simulink model "sampleModel20"  (R2021a)
settings: Solver=VariableStepAuto  StartTime=0.0  StopTime=10.0  RelTol=1e-3
undefined symbols (not defined in the file): DiscIntNeverNeededParam, magnitude, Newton, Raphson
libraries: simulink x274, pid_lib x17
(part 8 of 16)

== system sampleModel20/cfblk97/cfblk4/cfblk4 ==
  cfblk1 : Inport
  cfblk14 : Inport  Port=2
  cfblk15 : Inport  Port=3
  cfblk16 : Inport  Port=4
  cfblk17 : Inport  Port=5
  cfblk10 : Subsystem
  cfblk11 : Subsystem
  cfblk12 : Subsystem
  cfblk13 : Subsystem
  cfblk{18..23} (6 alike) : Delay  SampleTime=1
  cfblk3 : Trigonometry
  cfblk4 : ComplexToMagnitudeAngle
  cfblk5 : simulink/Math Operations/Slider Gain  gain=1  low=0  high=2
  cfblk6 : simulink/Math Operations/Slider Gain  gain=1  low=0  high=2
  cfblk7 : Abs
  cfblk8 : Subsystem
  cfblk9 : Subsystem
  cfblk2 : Outport
  wires:
  cfblk1/1 -> cfblk7/1, cfblk12/4(cfblk7)
  cfblk6/1 -> cfblk10/1(cfblk1)
  cfblk4/1 -> cfblk8/1(cfblk1)
  cfblk4/2 -> cfblk6/1, cfblk10/5(cfblk10), cfblk11/5(cfblk9), cfblk11/9(cfblk13), cfblk10/7(cfblk12)
  cfblk7/1 -> cfblk5/1, cfblk10/6(cfblk11), cfblk11/7(cfblk11), cfblk9/3(cfblk6), cfblk11/10(cfblk14)
  cfblk16/1 -> cfblk2/1
  cfblk11/1(cfblk2) -> cfblk13/2(cfblk12)
  cfblk12/1(cfblk2) -> cfblk11/1(cfblk1)
  cfblk10/1(cfblk2) -> cfblk18/1, cfblk19/1
  cfblk3/1 -> cfblk11/2(cfblk6), cfblk9/7(cfblk10)
  cfblk15/1 -> cfblk8/2(cfblk6)
  cfblk12/2(cfblk9) -> cfblk4/1
  cfblk5/1 -> cfblk12/2(cfblk5), cfblk9/4(cfblk7)
  cfblk17/1 -> cfblk10/2(cfblk7), cfblk11/6(cfblk10), cfblk13/3(cfblk13), cfblk13/5(cfblk15)
  cfblk14/1 -> cfblk9/1(cfblk1), cfblk13/6(cfblk16), cfblk9/6(cfblk9)
  cfblk13/1(cfblk2) -> cfblk10/3(cfblk8)
  cfblk13/2(cfblk17) -> cfblk9/5(cfblk8), cfblk20/1
  cfblk8/1(cfblk2) -> cfblk9/2(cfblk5)
  cfblk8/2(cfblk7) -> cfblk3/1, cfblk13/4(cfblk14), cfblk11/8(cfblk12)
  cfblk9/3(cfblk12) -> cfblk10/4(cfblk9)
  cfblk18/1 -> cfblk12/1(cfblk1)
  cfblk19/1 -> cfblk12/5(cfblk8)
  cfblk20/1 -> cfblk11/4(cfblk8)
  cfblk9/1(cfblk2) -> cfblk21/1
  cfblk21/1 -> cfblk13/1(cfblk1)
  cfblk9/2(cfblk11) -> cfblk22/1
  cfblk22/1 -> cfblk11/3(cfblk7)
  cfblk9/4(cfblk13) -> cfblk23/1
  cfblk23/1 -> cfblk12/3(cfblk6)

== system sampleModel20/cfblk97/cfblk4/cfblk5 ==
  cfblk1 : Inport
  cfblk7 : Inport  Port=2
  cfblk8 : Inport  Port=3
  cfblk9 : Inport  Port=4
  cfblk10 : Inport  Port=5
  cfblk11 : Inport  Port=6
  cfblk12 : Inport  Port=7
  cfblk13 : Inport  Port=8
  cfblk14 : Inport  Port=9
  cfblk15 : Inport  Port=10
  cfblk3 : Rounding
  cfblk4 : MinMax  Inputs=2
  cfblk5 : Sum  Inputs=+-
  cfblk6 : Abs
  cfblk2 : Outport
  cfblk16 : Outport  Port=2
  cfblk17 : Outport  Port=3
  wires:
  cfblk7/1 -> cfblk6/1
  cfblk12/1 -> cfblk3/1
  cfblk6/1 -> cfblk5/1
  cfblk13/1 -> cfblk17/1
  cfblk10/1 -> cfblk5/2
  cfblk1/1 -> cfblk4/1
  cfblk11/1 -> cfblk2/1
  cfblk3/1 -> cfblk4/2
  cfblk4/1 -> cfblk16/1

== system sampleModel20/cfblk97/cfblk4/cfblk6 ==
  cfblk1 : Inport
  cfblk9 : Inport  Port=2
  cfblk{12..16} (5 alike) : Delay  SampleTime=1
  cfblk3 : Abs
  cfblk4 : Abs
  cfblk5 : simulink/Math Operations/MinMax Running Resettable  Function=min  vinit=0.0
  cfblk6 : Constant  Value=[-933538233.402793]  SampleTime=1
  cfblk7 : Subsystem
  cfblk8 : Subsystem
  cfblk2 : Outport
  cfblk10 : Outport  Port=2
  cfblk11 : Outport  Port=3
  wires:
  cfblk3/1 -> cfblk8/1(cfblk1), cfblk8/5(cfblk11)
  cfblk8/2(cfblk15) -> cfblk2/1
  cfblk6/1 -> cfblk5/1
  cfblk4/1 -> cfblk8/2(cfblk8), cfblk5/2, cfblk15/1, cfblk16/1
  cfblk7/1(cfblk2) -> cfblk8/3(cfblk9)
  cfblk7/2(cfblk13) -> cfblk3/1
  cfblk7/3(cfblk14) -> cfblk10/1
  cfblk5/1 -> cfblk8/6(cfblk12), cfblk8/7(cfblk13), cfblk8/8(cfblk14), cfblk13/1, cfblk14/1
  cfblk7/4(cfblk15) -> cfblk4/1
  cfblk9/1 -> cfblk8/4(cfblk10), cfblk7/5(cfblk10)
  cfblk1/1 -> cfblk7/3(cfblk8)
  cfblk7/5(cfblk16) -> cfblk11/1
  cfblk8/1(cfblk2) -> cfblk12/1
  cfblk12/1 -> cfblk7/1(cfblk1)
  cfblk13/1 -> cfblk7/2(cfblk7)
  cfblk14/1 -> cfblk7/7(cfblk12)
  cfblk15/1 -> cfblk7/4(cfblk9)
  cfblk16/1 -> cfblk7/6(cfblk11)

== system sampleModel20/cfblk100/cfblk11/cfblk7/cfblk4 ==
  cfblk1 : Inport
  cfblk9 : Inport  Port=2
  cfblk10 : Inport  Port=3
  cfblk11 : Inport  Port=4
  cfblk12 : Inport  Port=5
  cfblk13 : Inport  Port=6
  cfblk14 : Inport  Port=7
  cfblk15 : Inport  Port=8
  cfblk3 : Math  Operator=magnitude^2  SaturateOnIntegerOverflow=on
  cfblk4 : ComplexToRealImag
  cfblk5 : Gain  Gain=[-735360419.453945]
  cfblk6 : ComplexToMagnitudeAngle
  cfblk7 : MinMax
  cfblk8 : Sum  Inputs=+
  cfblk2 : Outport
  cfblk16 : Outport  Port=2
  cfblk17 : Outport  Port=3
  wires:
  cfblk14/1 -> cfblk7/1
  cfblk8/1 -> cfblk6/1
  cfblk15/1 -> cfblk16/1
  cfblk3/1 -> cfblk4/1
  cfblk13/1 -> cfblk17/1
  cfblk12/1 -> cfblk2/1
  cfblk9/1 -> cfblk5/1
  cfblk1/1 -> cfblk8/1
  cfblk6/1 -> cfblk3/1

== system sampleModel20/cfblk100/cfblk11/cfblk7/cfblk5 ==
  cfblk1 : Inport
  cfblk6 : Inport  Port=2
  cfblk7 : Inport  Port=3
  cfblk3 : Sum  Inputs=|++
  cfblk4 : simulink/Math Operations/MinMax Running Resettable  Function=min  vinit=0.0
  cfblk5 : MinMax
  cfblk2 : Outport
  cfblk8 : Outport  Port=2
  cfblk9 : Outport  Port=3
  cfblk10 : Outport  Port=4
  wires:
  cfblk3/1 -> cfblk2/1, cfblk4/1
  cfblk5/1 -> cfblk10/1
  cfblk4/1 -> cfblk5/1
  cfblk6/1 -> cfblk8/1, cfblk3/2
  cfblk1/1 -> cfblk9/1
  cfblk7/1 -> cfblk3/1, cfblk4/2

== system sampleModel20/cfblk100/cfblk11/cfblk7/cfblk6 ==
  cfblk1 : Inport
  cfblk10 : Inport  Port=2
  cfblk11 : Inport  Port=3
  cfblk12 : Inport  Port=4
  cfblk13 : Inport  Port=5
  cfblk3 : simulink/Math Operations/MinMax Running Resettable  Function=min  vinit=0.0
  cfblk4 : simulink/Math Operations/Slider Gain  gain=1  low=0  high=2
  cfblk5 : Sin  TimeSource=Use external signal  SampleTime=0
  cfblk6 : Squeeze
  cfblk7 : DotProduct  InputSameDT=on  OutDataTypeStr=Inherit: Inherit via internal rule
  cfblk8 : MinMax  Function=max  Inputs=3
  cfblk9 : Abs
  cfblk2 : Outport
  cfblk14 : Outport  Port=2
  wires:
  cfblk10/1 -> cfblk5/1
  cfblk11/1 -> cfblk2/1
  cfblk9/1 -> cfblk6/1
  cfblk5/1 -> cfblk4/1, cfblk8/3
  cfblk1/1 -> cfblk8/1
  cfblk3/1 -> cfblk7/1
  cfblk7/1 -> cfblk14/1
  cfblk4/1 -> cfblk9/1
  cfblk13/1 -> cfblk3/1
  cfblk8/1 -> cfblk3/2
  cfblk12/1 -> cfblk8/2
  cfblk6/1 -> cfblk7/2

== system sampleModel20/cfblk100/cfblk11/cfblk8/cfblk12 ==
  cfblk1 : Inport
  cfblk10 : Inport  Port=2
  cfblk11 : Inport  Port=3
  cfblk12 : Inport  Port=4
  cfblk13 : Inport  Port=5
  cfblk14 : Inport  Port=6
  Action Port : ActionPort  ActionPortLabel=if(u1 >= 0)
  cfblk3 : Polyval  Coefs=[ +2.081618890e-019, -1.441693666e-014, +4.719686976e-010, -8.536869453e-006, +1.621573104e-001, -8.087801117e+001 ]
  cfblk4 : UnaryMinus
  cfblk5 : Product  Inputs=**
  cfblk6 : Sqrt  SaturateOnIntegerOverflow=on
  cfblk7 : simulink/Math Operations/Slider Gain  gain=1  low=0  high=2
  cfblk8 : MinMax  Function=max
  cfblk9 : Sum  Inputs=|++
  cfblk2 : Outport
  cfblk15 : Outport  Port=2
  cfblk16 : Outport  Port=3
  wires:
  cfblk9/1 -> cfblk5/1
  cfblk6/1 -> cfblk7/1
  cfblk5/1 -> cfblk15/1
  cfblk1/1 -> cfblk5/2
  cfblk11/1 -> cfblk2/1
  cfblk4/1 -> cfblk6/1
  cfblk14/1 -> cfblk3/1
  cfblk7/1 -> cfblk9/1
  cfblk3/1 -> cfblk4/1
  cfblk12/1 -> cfblk16/1
  cfblk8/1 -> cfblk9/2
  cfblk13/1 -> cfblk8/1

== system sampleModel20/cfblk100/cfblk11/cfblk8/cfblk13 ==
  cfblk1 : Inport
  cfblk4 : Inport  Port=2
  cfblk5 : Inport  Port=3
  cfblk6 : Inport  Port=4
  cfblk7 : Inport  Port=5
  cfblk8 : Inport  Port=6
  cfblk9 : Inport  Port=7
  Action Port : ActionPort  ActionPortLabel=else
  cfblk3 : Squeeze
  cfblk2 : Outport
  wires:
  cfblk9/1 -> cfblk2/1
  cfblk7/1 -> cfblk3/1

== system sampleModel20/cfblk100/cfblk11/cfblk8/cfblk5 ==
  cfblk1 : Inport
  cfblk5 : Inport  Port=2
  cfblk6 : Inport  Port=3
  cfblk7 : Inport  Port=4
  cfblk3 : Bias  Bias=[-726491726.571453]
  cfblk4 : DotProduct  InputSameDT=on  OutDataTypeStr=Inherit: Inherit via internal rule
  cfblk2 : Outport
  cfblk8 : Outport  Port=2
  wires:
  cfblk1/1 -> cfblk2/1
  cfblk7/1 -> cfblk3/1
  cfblk3/1 -> cfblk8/1
  cfblk5/1 -> cfblk4/1
  cfblk6/1 -> cfblk4/2

== system sampleModel20/cfblk100/cfblk11/cfblk8/cfblk6 ==
  cfblk1 : Inport
  cfblk6 : Inport  Port=2
  cfblk7 : Inport  Port=3
  cfblk8 : Inport  Port=4
  cfblk9 : Inport  Port=5
  cfblk10 : Inport  Port=6
  cfblk11 : Inport  Port=7
  cfblk12 : Inport  Port=8
  cfblk13 : Inport  Port=9
  cfblk3 : Bias  Bias=[914019764.906986]
  cfblk4 : Sqrt  SaturateOnIntegerOverflow=on
  cfblk5 : Reshape
  cfblk2 : Outport
  wires:
  cfblk3/1 -> cfblk5/1
  cfblk9/1 -> cfblk4/1
  cfblk10/1 -> cfblk2/1
  cfblk8/1 -> cfblk3/1

== system sampleModel20/cfblk100/cfblk11/cfblk8/cfblk7 ==
  cfblk1 : Inport
  cfblk8 : Inport  Port=2
  cfblk9 : Inport  Port=3
  cfblk10 : Inport  Port=4
  cfblk11 : Inport  Port=5
  cfblk12 : Inport  Port=6
  cfblk3 : Product  Inputs=*
  cfblk4 : DotProduct  InputSameDT=on  OutDataTypeStr=Inherit: Inherit via internal rule
  cfblk5 : PermuteDimensions
  cfblk6 : ComplexToMagnitudeAngle
  cfblk7 : Rounding
  cfblk2 : Outport
  cfblk13 : Outport  Port=2
  cfblk14 : Outport  Port=3
  cfblk15 : Outport  Port=4
  cfblk16 : Outport  Port=5
  wires:
  cfblk12/1 -> cfblk7/1
  cfblk6/1 -> cfblk15/1
  cfblk11/1 -> cfblk13/1
  cfblk6/2 -> cfblk3/1
  cfblk1/1 -> cfblk14/1
  cfblk5/1 -> cfblk4/1
  cfblk7/1 -> cfblk6/1
  cfblk10/1 -> cfblk2/1
  cfblk8/1 -> cfblk16/1
  cfblk9/1 -> cfblk5/1
  cfblk3/1 -> cfblk4/2

== system sampleModel20/cfblk100/cfblk8/cfblk10/cfblk10 ==
  cfblk1 : Inport
  cfblk10 : Inport  Port=2
  cfblk11 : Inport  Port=3
  cfblk12 : Inport  Port=4
  cfblk13 : Inport  Port=5
  cfblk14 : Inport  Port=6
  cfblk15 : Delay  SampleTime=1
  cfblk3 : Rounding
  cfblk4 : simulink/Math Operations/MinMax Running Resettable  Function=min  vinit=0.0
  cfblk5 : Product  Inputs=*
  cfblk6 : Rounding
  cfblk7 : PermuteDimensions
  cfblk8 : Sum  Inputs=+-
  cfblk9 : Product
  cfblk2 : Outport
  wires:
  cfblk7/1 -> cfblk8/1
  cfblk12/1 -> cfblk4/1
  cfblk3/1 -> cfblk6/1
  cfblk6/1 -> cfblk9/1
  cfblk8/1 -> cfblk2/1
  cfblk5/1 -> cfblk4/2
  cfblk4/1 -> cfblk8/2
  cfblk1/1 -> cfblk5/1
  cfblk13/1 -> cfblk7/1
  cfblk14/1 -> cfblk9/2
  cfblk9/1 -> cfblk15/1
  cfblk15/1 -> cfblk3/1

== system sampleModel20/cfblk100/cfblk8/cfblk7/cfblk6 ==
  cfblk1 : Inport
  cfblk12 : Inport  Port=2
  cfblk13 : Inport  Port=3
  cfblk14 : Inport  Port=4
  cfblk15 : Inport  Port=5
  cfblk16 : Inport  Port=6
  cfblk10 : Polyval  Coefs=[ +2.081618890e-019, -1.441693666e-014, +4.719686976e-010, -8.536869453e-006, +1.621573104e-001, -8.087801117e+001 ]
  cfblk11 : Rounding
  cfblk3 : Delay  ShowEnablePort=on  SampleTime=1
      settings: InputPortMap=u0,e6
  cfblk4 : Signum
  cfblk5 : Sum
  cfblk6 : Reshape
  cfblk7 : Signum
  cfblk8 : Product  Inputs=*
  cfblk9 : Gain  Gain=[-652010099.708883]
  cfblk2 : Outport
  cfblk17 : Outport  Port=2
  wires:
  cfblk11/1 -> cfblk7/1
  cfblk14/1 -> cfblk11/1
  cfblk3/1 -> cfblk2/1
  cfblk12/1 -> cfblk6/1
  cfblk10/1 -> cfblk4/1
  cfblk7/1 -> cfblk8/1
  cfblk4/1 -> cfblk9/1
  cfblk13/1 -> cfblk5/1
  cfblk6/1 -> cfblk3/1
  cfblk9/1 -> cfblk5/2
  cfblk1/1 -> cfblk3/2
  cfblk16/1 -> cfblk10/1
  cfblk15/1 -> cfblk17/1

== system sampleModel20/cfblk100/cfblk8/cfblk8/cfblk7 ==
  cfblk1 : Inport
  cfblk10 : Inport  Port=2
  cfblk11 : Inport  Port=3
  cfblk12 : Inport  Port=4
  cfblk13 : Inport  Port=5
  cfblk14 : Inport  Port=6
  cfblk15 : Inport  Port=7
  cfblk3 : Sum  Inputs=+
  cfblk4 : ComplexToRealImag
  cfblk5 : Reshape
  cfblk6 : MinMax  Inputs=3
  cfblk7 : ComplexToMagnitudeAngle
  cfblk8 : Rounding
  cfblk9 : ComplexToRealImag
  cfblk2 : Outport
  cfblk16 : Outport  Port=2
  wires:
  cfblk14/1 -> cfblk6/1
  cfblk8/1 -> cfblk16/1
  cfblk9/1 -> cfblk3/1
  cfblk7/1 -> cfblk8/1
  cfblk4/1 -> cfblk7/1
  cfblk11/1 -> cfblk5/1
  cfblk13/1 -> cfblk9/1
  cfblk9/2 -> cfblk4/1
  cfblk6/1 -> cfblk2/1
  cfblk7/2 -> cfblk6/2
  cfblk1/1 -> cfblk6/3

== system sampleModel20/cfblk100/cfblk8/cfblk8/cfblk8 ==
  cfblk1 : Inport
  cfblk6 : Inport  Port=2
  cfblk7 : Inport  Port=3
  cfblk8 : Inport  Port=4
  cfblk9 : Inport  Port=5
  cfblk10 : Inport  Port=6
  cfblk3 : DotProduct  InputSameDT=on  OutDataTypeStr=Inherit: Inherit via internal rule
  cfblk4 : Sum  Inputs=+-
  cfblk5 : Bias  Bias=[732439637.067177]
  cfblk2 : Outport
  cfblk11 : Outport  Port=2
  wires:
  cfblk1/1 -> cfblk2/1
  cfblk10/1 -> cfblk4/1
  cfblk8/1 -> cfblk4/2
  cfblk6/1 -> cfblk11/1
  cfblk4/1 -> cfblk5/1
  cfblk5/1 -> cfblk3/1
  cfblk7/1 -> cfblk3/2

== system sampleModel20/cfblk100/cfblk8/cfblk9/cfblk6 ==
  cfblk1 : Inport
  cfblk9 : Inport  Port=2
  cfblk10 : Inport  Port=3
  cfblk11 : Inport  Port=4
  cfblk12 : Inport  Port=5
  cfblk13 : Inport  Port=6
  cfblk14 : Inport  Port=7
  cfblk15 : Inport  Port=8
  cfblk16 : Inport  Port=9
  cfblk3 : pid_lib/PID Controller (2DOF)  Controller=PID  Form=Parallel  TimeDomain=Discrete-time  UseExternalTs=off  SampleTime=1  IntegratorMethod=Forward Euler  FilterMethod=Forward Euler  ControllerParametersSource=internal  P=1  I=1  D=0  UseFilter=on  N=100  b=1  c=1  TunerSelectOption=Transfer Function Based (PID Tuner App)  InitialConditionSource=internal  InitialConditionForIntegrator=0  InitialConditionForFilter=0  DifferentiatorICPrevScaledInput=0  ExternalReset=none  TrackingMode=off  Kt=1  LimitOutput=off  SatLimitsSource=internal  UpperSaturationLimit=inf  LowerSaturationLimit=-inf  LinearizeAsGain=off  AntiWindupMode=none  Kb=1  POutMin=[]  POutMax=[]  IOutMin=[]  IOutMax=[]  DOutMin=[]  DOutMax=[]  NOutMin=[]  NOutMax=[]  bOutMin=[]  bOutMax=[]  cOutMin=[]  cOutMax=[]  SumOutMin=[]  SumOutMax=[]  SaturationOutMin=[]  SaturationOutMax=[]  PParamMin=[]  PParamMax=[]  IParamMin=[]  IParamMax=[]  DParamMin=[]  DParamMax=[]  NParamMin=[]  NParamMax=[]  bParamMin=[]  bParamMax=[]  cParamMin=[]  cParamMax=[]  KbParamMin=[]  KbParamMax=[]  KtParamMin=[]  KtParamMax=[]  KbOutMin=[]  KbOutMax=[]  KtOutMin=[]  KtOutMax=[]  IntegratorOutMin=[]  IntegratorOutMax=[]  FilterOutMin=[]  FilterOutMax=[]  SumI1OutMin=[]  SumI1OutMax=[]  SumI2OutMin=[]  SumI2OutMax=[]  SumI3OutMin=[]  SumI3OutMax=[]  SumI4OutMin=[]  SumI4OutMax=[]  SumDOutMin=[]  SumDOutMax=[]  Sum1OutMin=[]  Sum1OutMax=[]  Sum2OutMin=[]  Sum2OutMax=[]  Sum3OutMin=[]  Sum3OutMax=[]  DifferentiatorOutMin=[]  DifferentiatorOutMax=[]  FilterDiffOutCoefMin=[]  FilterDiffOutCoefMax=[]  ReciprocalOutMin=[]  ReciprocalOutMax=[]  SumDenOutMin=[]  SumDenOutMax=[]  SumNumOutMin=[]  SumNumOutMax=[]  DivideOutMin=[]  DivideOutMax=[]  UdiffTsProdOutMin=[]  UdiffTsProdOutMax=[]  NTsProdOutMin=[]  NTsProdOutMax=[]  UintegralTsProdOutMin=[]  UintegralTsProdOutMax=[]  UngainTsProdOutMin=[]  UngainTsProdOutMax=[]  IntegratorContinuousStateAttributes=''  IntegratorStateMustResolveToSignalObject=off  IntegratorRTWStateStorageClass=Auto  FilterContinuousStateAttributes=''  FilterStateMustResolveToSignalObject=off  FilterRTWStateStorageClass=Auto  ParallelPVariant=InternalParameters  IdealPVariant=Disabled  IVariant=InternalParameters  DVariant=InternalParameters  bVariant=InternalParameters  cVariant=InternalParameters  IntegratorVariant=Discrete  SatVariant=Disabled  AWVariant=Passthrough  PCopyVariant=Disabled  TRVariant=Disabled  FdbkBlocksVariant=Forward  IdealPFdbkVariant=Disabled  SatFdbkVariant=Disabled  DerivativeFilterVariant=ForwardEulerFilter  NVariant=InternalParameters  NCopyVariant=Disabled  FilterICVariant=InternalICsFilter  IntegratorICVariant=InternalICs  ExternalResetVariant=Disabled  TRSumVariant=Passthrough  SumFdbkVariant=Disabled  SumVariant=Sum_PID  TsampFilterVariant=InternalTs  TsampNgainVariant=Passthrough  TsampIntegralVariant=Passthrough  ExternalSaturationOutDataTypeStr=Inherit: Same as second input
      settings: SourceProductBaseCode=SL
  cfblk4 : DiscreteTransferFcn  SampleTime=1
  cfblk5 : Sum  Inputs=+-
  cfblk6 : ComplexToRealImag
  cfblk7 : Product  Inputs=*
  cfblk8 : DotProduct  InputSameDT=on  OutDataTypeStr=Inherit: Inherit via internal rule
  cfblk2 : Outport
  cfblk17 : Outport  Port=2
  wires:
  cfblk6/1 -> cfblk17/1
  cfblk5/1 -> cfblk6/1
  cfblk13/1 -> cfblk5/1
  cfblk14/1 -> cfblk5/2
  cfblk7/1 -> cfblk8/1
  cfblk6/2 -> cfblk3/1
  cfblk1/1 -> cfblk3/2
  cfblk10/1 -> cfblk8/2
  cfblk3/1 -> cfblk4/1
  cfblk11/1 -> cfblk7/1
  cfblk9/1 -> cfblk2/1

== system sampleModel20/cfblk100/cfblk8/cfblk9/cfblk7 ==
  cfblk1 : Inport
  cfblk7 : Inport  Port=2
  cfblk8 : Inport  Port=3
  cfblk3 : Product  Inputs=*
  cfblk4 : ComplexToMagnitudeAngle
  cfblk5 : MinMax
  cfblk6 : simulink/Math Operations/Slider Gain  gain=1  low=0  high=2
  cfblk2 : Outport
  wires:
  cfblk8/1 -> cfblk6/1
  cfblk5/1 -> cfblk2/1
  cfblk1/1 -> cfblk4/1
  cfblk4/1 -> cfblk5/1
  cfblk7/1 -> cfblk3/1

== system sampleModel20/cfblk100/cfblk8/cfblk9/cfblk8 ==
  cfblk1 : Inport
  cfblk14 : Inport  Port=2
  cfblk15 : Inport  Port=3
  cfblk10 : Assignment  DiagnosticForDimensions=Warning  IndexOptions=Index vector (dialog)  Indices=1  OutputSizes=1
  cfblk11 : Sum  Inputs=+-
  cfblk12 : Sum
  cfblk13 : Sqrt  Operator=rSqrt  AlgorithmType=Newton-Raphson  SaturateOnIntegerOverflow=on
  cfblk18 : Delay  SampleTime=1
  cfblk19 : Delay  SampleTime=1
  cfblk20 : Delay  SampleTime=1
  cfblk3 : ComplexToRealImag
  cfblk4 : Sin  TimeSource=Use external signal  SampleTime=0
  cfblk5 : Abs
  cfblk6 : Sum  Inputs=|++
  cfblk7 : Gain  Gain=[-418794012.484760]
  cfblk8 : Sum  Inputs=+-
  cfblk9 : Sqrt  Operator=rSqrt  AlgorithmType=Newton-Raphson  SaturateOnIntegerOverflow=on
  cfblk2 : Outport
  cfblk16 : Outport  Port=2
  cfblk17 : Outport  Port=3
  wires:
  cfblk5/1 -> cfblk12/1
  cfblk3/1 -> cfblk2/1
  cfblk4/1 -> cfblk9/1
  cfblk14/1 -> cfblk3/1, cfblk5/1
  cfblk3/2 -> cfblk6/1
  cfblk6/1 -> cfblk11/2
  cfblk9/1 -> cfblk6/2, cfblk19/1
  cfblk11/1 -> cfblk12/2
  cfblk10/1 -> cfblk13/1
  cfblk12/1 -> cfblk8/1
  cfblk1/1 -> cfblk16/1
  cfblk15/1 -> cfblk7/1
  cfblk13/1 -> cfblk17/1, cfblk20/1
  cfblk7/1 -> cfblk10/1, cfblk8/2
  cfblk8/1 -> cfblk18/1
  cfblk18/1 -> cfblk11/1
  cfblk19/1 -> cfblk4/1
  cfblk20/1 -> cfblk10/2

== system sampleModel20/cfblk100/cfblk9/cfblk6/cfblk10 ==
  cfblk1 : Inport
  cfblk7 : Inport  Port=2
  cfblk8 : Inport  Port=3
  cfblk9 : Inport  Port=4
  cfblk10 : Inport  Port=5
  cfblk11 : Inport  Port=6
  cfblk12 : Delay  SampleTime=1
  cfblk3 : Sin  TimeSource=Use external signal  SampleTime=0
  cfblk4 : ComplexToRealImag
  cfblk5 : Trigonometry
  cfblk6 : Sqrt  SaturateOnIntegerOverflow=on
  cfblk2 : Outport
  wires:
  cfblk7/1 -> cfblk2/1
  cfblk4/1 -> cfblk6/1
  cfblk4/2 -> cfblk3/1
  cfblk10/1 -> cfblk5/1
  cfblk6/1 -> cfblk12/1
  cfblk12/1 -> cfblk4/1

== system sampleModel20/cfblk100/cfblk9/cfblk6/cfblk11 ==
  cfblk1 : Inport
  cfblk11 : Inport  Port=2
  cfblk12 : Inport  Port=3
  cfblk13 : Inport  Port=4
  cfblk14 : Inport  Port=5
  cfblk15 : Inport  Port=6
  cfblk16 : Inport  Port=7
  cfblk17 : Inport  Port=8
  cfblk10 : Sin  TimeSource=Use external signal  SampleTime=0
  cfblk3 : DiscreteZeroPole  Poles=[0 0.5]  Gain=1
  cfblk4 : Product  Inputs=**
  cfblk5 : Sqrt  Operator=rSqrt  AlgorithmType=Newton-Raphson  SaturateOnIntegerOverflow=on
  cfblk6 : Product
  cfblk7 : Product  Inputs=*
  cfblk8 : simulink/Math Operations/MinMax Running Resettable  Function=min  vinit=0.0
  cfblk9 : Gain  Gain=[-112072840.824712]
  cfblk2 : Outport
  wires:
  cfblk7/1 -> cfblk9/1
  cfblk13/1 -> cfblk10/1
  cfblk6/1 -> cfblk8/1
  cfblk11/1 -> cfblk8/2
  cfblk14/1 -> cfblk2/1
  cfblk12/1 -> cfblk3/1
  cfblk15/1 -> cfblk6/1
  cfblk3/1 -> cfblk5/1
  cfblk17/1 -> cfblk4/1
  cfblk5/1 -> cfblk7/1
  cfblk10/1 -> cfblk4/2
  cfblk1/1 -> cfblk6/2

== system sampleModel20/cfblk100/cfblk9/cfblk6/cfblk12 ==
  cfblk1 : Inport
  cfblk5 : Inport  Port=2
  cfblk6 : Inport  Port=3
  cfblk7 : Inport  Port=4
  cfblk3 : Sum  Inputs=+
  cfblk4 : Product
  cfblk2 : Outport
  cfblk8 : Outport  Port=2
  wires:
  cfblk3/1 -> cfblk4/1
  cfblk4/1 -> cfblk2/1
  cfblk7/1 -> cfblk8/1
  cfblk5/1 -> cfblk3/1
  cfblk1/1 -> cfblk4/2

== system sampleModel20/cfblk100/cfblk9/cfblk6/cfblk13 ==
  cfblk1 : Inport
  cfblk12 : Inport  Port=2
  cfblk13 : Inport  Port=3
  cfblk14 : Inport  Port=4
  cfblk15 : Inport  Port=5
  cfblk10 : Math  Operator=rem  SaturateOnIntegerOverflow=on
  cfblk11 : Squeeze
  cfblk3 : Sum  Inputs=--
  cfblk4 : Polyval  Coefs=[ +2.081618890e-019, -1.441693666e-014, +4.719686976e-010, -8.536869453e-006, +1.621573104e-001, -8.087801117e+001 ]
  cfblk5 : Sin  TimeSource=Use external signal  SampleTime=0
  cfblk6 : Reshape
  cfblk7 : simulink/Math Operations/Slider Gain  gain=1  low=0  high=2
  cfblk8 : UnaryMinus
  cfblk9 : PermuteDimensions
  cfblk2 : Outport
  cfblk16 : Outport  Port=2
  wires:
  cfblk5/1 -> cfblk3/1
  cfblk6/1 -> cfblk2/1
  cfblk11/1 -> cfblk3/2
  cfblk10/1 -> cfblk5/1
  cfblk4/1 -> cfblk11/1
  cfblk8/1 -> cfblk10/1
  cfblk7/1 -> cfblk4/1
  cfblk12/1 -> cfblk8/1
  cfblk3/1 -> cfblk16/1
  cfblk14/1 -> cfblk6/1
  cfblk9/1 -> cfblk7/1
  cfblk15/1 -> cfblk10/2
  cfblk1/1 -> cfblk9/1

== system sampleModel20/cfblk100/cfblk9/cfblk7/cfblk5 ==
  cfblk1 : Inport
  cfblk5 : Inport  Port=2
  cfblk6 : Inport  Port=3
  cfblk7 : Inport  Port=4
  cfblk8 : Inport  Port=5
  cfblk9 : Inport  Port=6
  cfblk10 : Inport  Port=7
  cfblk11 : Inport  Port=8
  cfblk12 : Inport  Port=9
  cfblk13 : Inport  Port=10
  cfblk14 : Inport  Port=11
  cfblk15 : Inport  Port=12
  cfblk16 : Inport  Port=13
  cfblk3 : Signum
  cfblk4 : Sin  TimeSource=Use external signal  SampleTime=0
  cfblk2 : Outport
  cfblk17 : Outport  Port=2
  wires:
  cfblk4/1 -> cfblk3/1
  cfblk12/1 -> cfblk2/1
  cfblk16/1 -> cfblk4/1
  cfblk3/1 -> cfblk17/1

== system sampleModel20/cfblk100/cfblk9/cfblk7/cfblk6 ==
  cfblk1 : Inport
  cfblk9 : Inport  Port=2
  cfblk10 : Inport  Port=3
  cfblk11 : Inport  Port=4
  cfblk12 : Inport  Port=5
  cfblk13 : Inport  Port=6
  cfblk14 : Inport  Port=7
  cfblk15 : Inport  Port=8
  cfblk16 : Inport  Port=9
  cfblk17 : Inport  Port=10
  cfblk3 : Bias  Bias=[318969585.120855]
  cfblk4 : Gain  Gain=[263061233.365778]
  cfblk5 : DotProduct  InputSameDT=on  OutDataTypeStr=Inherit: Inherit via internal rule
  cfblk6 : Rounding
  cfblk7 : Product  Inputs=*
  cfblk8 : Sqrt  SaturateOnIntegerOverflow=on
  cfblk2 : Outport
  wires:
  cfblk14/1 -> cfblk7/1
  cfblk17/1 -> cfblk5/1
  cfblk6/1 -> cfblk3/1
  cfblk8/1 -> cfblk5/2
  cfblk1/1 -> cfblk4/1
  cfblk16/1 -> cfblk2/1
  cfblk4/1 -> cfblk6/1
  cfblk3/1 -> cfblk8/1

== system sampleModel20/cfblk100/cfblk9/cfblk7/cfblk7 ==
  cfblk1 : Inport
  cfblk11 : Inport  Port=2
  cfblk12 : Inport  Port=3
  cfblk13 : Inport  Port=4
  cfblk14 : Inport  Port=5
  cfblk15 : Inport  Port=6
  cfblk10 : Sum  Inputs=+
  cfblk3 : Reshape
  cfblk4 : Sum  Inputs=|++
  cfblk5 : Polyval  Coefs=[ +2.081618890e-019, -1.441693666e-014, +4.719686976e-010, -8.536869453e-006, +1.621573104e-001, -8.087801117e+001 ]
  cfblk6 : UnaryMinus
  cfblk7 : Sum  Inputs=|++
  cfblk8 : Sum  Inputs=-+
  cfblk9 : Assignment  DiagnosticForDimensions=Warning  IndexOptions=Index vector (dialog)  Indices=1  OutputSizes=1
  cfblk2 : Outport
  cfblk16 : Outport  Port=2
  cfblk17 : Outport  Port=3
  wires:
  cfblk12/1 -> cfblk6/1
  cfblk10/1 -> cfblk8/1
  cfblk8/1 -> cfblk16/1
  cfblk13/1 -> cfblk7/1
  cfblk7/1 -> cfblk10/1
  cfblk15/1 -> cfblk9/1
  cfblk1/1 -> cfblk3/1
  cfblk5/1 -> cfblk8/2
  cfblk9/1 -> cfblk17/1
  cfblk6/1 -> cfblk4/1
  cfblk14/1 -> cfblk2/1
  cfblk3/1 -> cfblk5/1
  cfblk4/1 -> cfblk9/2
  cfblk11/1 -> cfblk7/2, cfblk4/2

== system sampleModel20/cfblk100/cfblk9/cfblk7/cfblk8 ==
  cfblk1 : Inport
  cfblk7 : Inport  Port=2
  cfblk8 : Inport  Port=3
  cfblk9 : Inport  Port=4
  cfblk10 : Inport  Port=5
  cfblk3 : Polyval  Coefs=[ +2.081618890e-019, -1.441693666e-014, +4.719686976e-010, -8.536869453e-006, +1.621573104e-001, -8.087801117e+001 ]
  cfblk4 : ComplexToRealImag
  cfblk5 : ComplexToRealImag
  cfblk6 : Bias  Bias=[528797732.051114]
  cfblk2 : Outport
  cfblk11 : Outport  Port=2
  cfblk12 : Outport  Port=3
  wires:
  cfblk3/1 -> cfblk2/1
  cfblk7/1 -> cfblk4/1
  cfblk1/1 -> cfblk11/1
  cfblk9/1 -> cfblk3/1
  cfblk6/1 -> cfblk12/1
  cfblk8/1 -> cfblk5/1
  cfblk10/1 -> cfblk6/1

== system sampleModel20/cfblk100/cfblk9/cfblk7/cfblk9 ==
  cfblk1 : Inport
  cfblk12 : Inport  Port=2
  cfblk13 : Inport  Port=3
  cfblk14 : Inport  Port=4
  cfblk10 : ComplexToMagnitudeAngle
  cfblk11 : Reshape
  cfblk3 : ComplexToRealImag
  cfblk4 : Sum  Inputs=|++
  cfblk5 : Trigonometry
  cfblk6 : ComplexToRealImag
  cfblk7 : Trigonometry
  cfblk8 : Product  Inputs=**
  cfblk9 : Squeeze
  cfblk2 : Outport
  wires:
  cfblk13/1 -> cfblk3/1
  cfblk8/1 -> cfblk2/1
  cfblk9/1 -> cfblk7/1
  cfblk1/1 -> cfblk8/1
  cfblk3/1 -> cfblk5/1
  cfblk6/1 -> cfblk9/1
  cfblk3/2 -> cfblk8/2
  cfblk7/1 -> cfblk11/1
  cfblk12/1 -> cfblk4/1
  cfblk4/1 -> cfblk6/1
  cfblk10/1 -> cfblk4/2
  cfblk5/1 -> cfblk10/1

== system sampleModel20/cfblk100/cfblk9/cfblk8/cfblk6 ==
  cfblk1 : Inport
  cfblk3 : Inport  Port=2
  cfblk4 : Inport  Port=3
  cfblk5 : Inport  Port=4
  cfblk6 : Inport  Port=5
  cfblk7 : Inport  Port=6
  cfblk8 : Inport  Port=7
  cfblk9 : Inport  Port=8
  cfblk10 : Inport  Port=9
  cfblk2 : Outport
  wires:
  cfblk5/1 -> cfblk2/1

== system sampleModel20/cfblk100/cfblk9/cfblk8/cfblk7 ==
  cfblk1 : Inport
  cfblk7 : Inport  Port=2
  cfblk8 : Inport  Port=3
  cfblk9 : Inport  Port=4
  cfblk10 : Inport  Port=5
  cfblk11 : Inport  Port=6
  cfblk12 : Inport  Port=7
  cfblk14 : Delay  SampleTime=1
  cfblk3 : Sum  Inputs=+-
  cfblk4 : Product  Inputs=**
  cfblk5 : Sum  Inputs=|++
  cfblk6 : ComplexToMagnitudeAngle
  cfblk2 : Outport
  cfblk13 : Outport  Port=2
  wires:
  cfblk7/1 -> cfblk6/1
  cfblk4/1 -> cfblk5/1
  cfblk1/1 -> cfblk2/1
  cfblk12/1 -> cfblk3/1
  cfblk11/1 -> cfblk3/2
  cfblk3/1 -> cfblk13/1
  cfblk10/1 -> cfblk5/2
  cfblk6/1 -> cfblk4/2
  cfblk5/1 -> cfblk14/1
  cfblk14/1 -> cfblk4/1

== system sampleModel20/cfblk100/cfblk9/cfblk9/cfblk10 ==
  cfblk1 : Inport
  cfblk8 : Inport  Port=2
  cfblk9 : Inport  Port=3
  cfblk10 : Inport  Port=4
  cfblk11 : Inport  Port=5
  cfblk12 : Inport  Port=6
  cfblk13 : Inport  Port=7
  cfblk14 : Inport  Port=8
  cfblk15 : Inport  Port=9
  cfblk16 : Inport  Port=10
  cfblk17 : Inport  Port=11
  cfblk3 : ComplexToRealImag
  cfblk4 : Sum  Inputs=--
  cfblk5 : Bias  Bias=[-305823638.469442]
  cfblk6 : Polyval  Coefs=[ +2.081618890e-019, -1.441693666e-014, +4.719686976e-010, -8.536869453e-006, +1.621573104e-001, -8.087801117e+001 ]
  cfblk7 : Sum  Inputs=-+
  cfblk2 : Outport
  wires:
  cfblk9/1 -> cfblk6/1
  cfblk13/1 -> cfblk5/1
  cfblk16/1 -> cfblk7/1
  cfblk4/1 -> cfblk7/2
  cfblk10/1 -> cfblk2/1
  cfblk15/1 -> cfblk4/1
  cfblk5/1 -> cfblk4/2
  cfblk6/1 -> cfblk3/1

== system sampleModel20/cfblk100/cfblk9/cfblk9/cfblk6 ==
  cfblk1 : Inport
  cfblk4 : Inport  Port=2
  cfblk5 : Inport  Port=3
  cfblk6 : Inport  Port=4
  cfblk7 : Inport  Port=5
  cfblk8 : Inport  Port=6
  cfblk9 : Inport  Port=7
  cfblk10 : Inport  Port=8
  cfblk3 : Sum  Inputs=+-
  cfblk2 : Outport
  cfblk11 : Outport  Port=2
  wires:
  cfblk1/1 -> cfblk2/1
  cfblk4/1 -> cfblk3/1
  cfblk9/1 -> cfblk3/2
  cfblk8/1 -> cfblk11/1

== system sampleModel20/cfblk100/cfblk9/cfblk9/cfblk7 ==
  cfblk1 : Inport
  cfblk11 : Inport  Port=2
  cfblk10 : simulink/Math Operations/Slider Gain  gain=1  low=0  high=2
  cfblk13 : Delay  SampleTime=1
  cfblk3 : Rounding
  cfblk4 : Product  Inputs=**
  cfblk5 : Signum
  cfblk6 : DotProduct  InputSameDT=on  OutDataTypeStr=Inherit: Inherit via internal rule
  cfblk7 : Sqrt  SaturateOnIntegerOverflow=on
  cfblk8 : Sin  TimeSource=Use external signal  SampleTime=0
  cfblk9 : Sin  TimeSource=Use external signal  SampleTime=0
  cfblk2 : Outport
  cfblk12 : Outport  Port=2
  wires:
  cfblk5/1 -> cfblk9/1, cfblk6/2
  cfblk4/1 -> cfblk5/1
  cfblk1/1 -> cfblk10/1
  cfblk8/1 -> cfblk7/1
  cfblk11/1 -> cfblk12/1, cfblk3/1
  cfblk10/1 -> cfblk4/1
  cfblk6/1 -> cfblk8/1
  cfblk9/1 -> cfblk2/1
  cfblk3/1 -> cfblk4/2
  cfblk7/1 -> cfblk13/1
  cfblk13/1 -> cfblk6/1

== system sampleModel20/cfblk100/cfblk9/cfblk9/cfblk8 ==
  cfblk1 : Inport
  cfblk9 : Inport  Port=2
  cfblk10 : Inport  Port=3
  cfblk11 : Inport  Port=4
  cfblk12 : Inport  Port=5
  cfblk13 : Inport  Port=6
  cfblk14 : Inport  Port=7
  cfblk15 : Inport  Port=8
  cfblk16 : Inport  Port=9
  cfblk17 : Inport  Port=10
  cfblk3 : simulink/Discrete/Transfer Fcn Lead or Lag  PoleZ=0.95  ZeroZ=0.75  ICPrevOutput=0.0  ICPrevInput=0.0  DoSatur=off
      settings: SourceProductBaseCode=SL
  cfblk4 : Sum  Inputs=+-
  cfblk5 : Assignment  DiagnosticForDimensions=Warning  IndexOptions=Index vector (dialog)  Indices=1  OutputSizes=1
  cfblk6 : Squeeze
  cfblk7 : Math  Operator=magnitude^2  SaturateOnIntegerOverflow=on
  cfblk8 : ComplexToMagnitudeAngle
  cfblk2 : Outport
  wires:
  cfblk17/1 -> cfblk5/1
  cfblk5/1 -> cfblk3/1
  cfblk6/1 -> cfblk8/1
  cfblk3/1 -> cfblk4/1
  cfblk4/1 -> cfblk6/1
  cfblk16/1 -> cfblk2/1
  cfblk9/1 -> cfblk4/2
  cfblk1/1 -> cfblk5/2
  cfblk13/1 -> cfblk7/1

== system sampleModel20/cfblk100/cfblk9/cfblk9/cfblk9 ==
  cfblk1 : Inport
  cfblk7 : Inport  Port=2
  cfblk8 : Inport  Port=3
  cfblk9 : Inport  Port=4
  cfblk10 : Inport  Port=5
  cfblk11 : Inport  Port=6
  cfblk3 : Product  Inputs=*
  cfblk4 : simulink/Math Operations/MinMax Running Resettable  Function=min  vinit=0.0
  cfblk5 : Gain  Gain=[-892001897.910358]
  cfblk6 : Abs
  cfblk2 : Outport
  cfblk12 : Outport  Port=2
  cfblk13 : Outport  Port=3
  wires:
  cfblk6/1 -> cfblk12/1
  cfblk1/1 -> cfblk2/1
  cfblk7/1 -> cfblk4/1
  cfblk3/1 -> cfblk6/1
  cfblk10/1 -> cfblk4/2
  cfblk9/1 -> cfblk13/1
  cfblk4/1 -> cfblk5/1
  cfblk11/1 -> cfblk3/1

== system sampleModel20/cfblk77/cfblk10/cfblk6/cfblk4 ==
  cfblk1 : Inport
  cfblk10 : Inport  Port=2
  cfblk11 : Inport  Port=3
  cfblk12 : Inport  Port=4
  cfblk3 : Sin  TimeSource=Use external signal  SampleTime=0
  cfblk4 : simulink/Math Operations/Slider Gain  gain=1  low=0  high=2
  cfblk5 : Product
  cfblk6 : UnaryMinus
  cfblk7 : Sqrt  SaturateOnIntegerOverflow=on
  cfblk8 : Signum
  cfblk9 : Product  Inputs=**
  cfblk2 : Outport
  wires:
  cfblk11/1 -> cfblk5/1
  cfblk12/1 -> cfblk6/1
  cfblk7/1 -> cfblk8/1
  cfblk6/1 -> cfblk7/1
  cfblk4/1 -> cfblk5/2
  cfblk3/1 -> cfblk2/1
  cfblk9/1 -> cfblk4/1
  cfblk8/1 -> cfblk9/1
  cfblk5/1 -> cfblk3/1
  cfblk1/1 -> cfblk9/2

== system sampleModel20/cfblk77/cfblk10/cfblk6/cfblk5 ==
  cfblk1 : Inport
  cfblk5 : Inport  Port=2
  cfblk6 : Inport  Port=3
  cfblk7 : Inport  Port=4
  cfblk3 : Product  Inputs=**
  cfblk4 : Sum  Inputs=|++
  cfblk2 : Outport
  wires:
  cfblk7/1 -> cfblk2/1
  cfblk6/1 -> cfblk4/1
  cfblk1/1 -> cfblk3/1
  cfblk5/1 -> cfblk4/2
  cfblk4/1 -> cfblk3/2

== system sampleModel20/cfblk77/cfblk10/cfblk6/cfblk6 ==
  cfblk1 : Inport
  cfblk5 : Inport  Port=2
  cfblk6 : Inport  Port=3
  cfblk7 : Inport  Port=4
  cfblk8 : Inport  Port=5
  cfblk9 : Inport  Port=6
  cfblk10 : Inport  Port=7
  cfblk3 : Polyval  Coefs=[ +2.081618890e-019, -1.441693666e-014, +4.719686976e-010, -8.536869453e-006, +1.621573104e-001, -8.087801117e+001 ]
  cfblk4 : Reshape
  cfblk2 : Outport
  wires:
  cfblk10/1 -> cfblk3/1
  cfblk8/1 -> cfblk4/1
  cfblk9/1 -> cfblk2/1

== system sampleModel20/cfblk77/cfblk10/cfblk7/cfblk10 ==
  cfblk1 : Inport
  cfblk12 : Inport  Port=2
  cfblk13 : Inport  Port=3
  cfblk14 : Inport  Port=4
  cfblk15 : Inport  Port=5
  cfblk16 : Inport  Port=6
  cfblk10 : simulink/Math Operations/Slider Gain  gain=1  low=0  high=2
  cfblk11 : Math  Operator=rem  SaturateOnIntegerOverflow=on
  cfblk3 : UnaryMinus
  cfblk4 : Sqrt  SaturateOnIntegerOverflow=on
  cfblk5 : Squeeze
  cfblk6 : Sqrt  Operator=rSqrt  AlgorithmType=Newton-Raphson  SaturateOnIntegerOverflow=on
  cfblk7 : Reshape
  cfblk8 : UnaryMinus
  cfblk9 : Sum  Inputs=+
  cfblk2 : Outport
  wires:
  cfblk5/1 -> cfblk9/1
  cfblk13/1 -> cfblk5/1
  cfblk9/1 -> cfblk6/1
  cfblk15/1 -> cfblk10/1
  cfblk6/1 -> cfblk4/1
  cfblk10/1 -> cfblk2/1
  cfblk1/1 -> cfblk8/1
  cfblk8/1 -> cfblk7/1
  cfblk16/1 -> cfblk3/1
  cfblk12/1 -> cfblk11/1
  cfblk7/1 -> cfblk11/2

== system sampleModel20/cfblk77/cfblk10/cfblk7/cfblk11 ==
  cfblk1 : Inport
  cfblk8 : Inport  Port=2
  cfblk9 : Inport  Port=3
  cfblk10 : Inport  Port=4
  cfblk11 : Inport  Port=5
  cfblk12 : Inport  Port=6
  cfblk13 : Inport  Port=7
  cfblk14 : Inport  Port=8
  cfblk3 : Bias  Bias=[569220854.138453]
  cfblk4 : DotProduct  InputSameDT=on  OutDataTypeStr=Inherit: Inherit via internal rule
  cfblk5 : Sum  Inputs=+
  cfblk6 : UnaryMinus
  cfblk7 : Signum
  cfblk2 : Outport
  wires:
  cfblk10/1 -> cfblk5/1
  cfblk12/1 -> cfblk7/1
  cfblk11/1 -> cfblk3/1
  cfblk8/1 -> cfblk6/1
  cfblk3/1 -> cfblk2/1
  cfblk1/1 -> cfblk4/1
  cfblk7/1 -> cfblk4/2

== system sampleModel20/cfblk77/cfblk10/cfblk7/cfblk12 ==
  cfblk1 : Inport
  cfblk7 : Inport  Port=2
  cfblk8 : Inport  Port=3
  cfblk9 : Inport  Port=4
  cfblk10 : Inport  Port=5
  cfblk11 : Inport  Port=6
  cfblk12 : Inport  Port=7
  cfblk13 : Inport  Port=8
  cfblk14 : Inport  Port=9
  cfblk3 : Sum  Inputs=|++
  cfblk4 : Sqrt  Operator=rSqrt  AlgorithmType=Newton-Raphson  SaturateOnIntegerOverflow=on
  cfblk5 : Abs
  cfblk6 : Squeeze
  cfblk2 : Outport
  cfblk15 : Outport  Port=2
  cfblk16 : Outport  Port=3
  cfblk17 : Outport  Port=4
  wires:
  cfblk10/1 -> cfblk5/1
  cfblk4/1 -> cfblk3/1
  cfblk3/1 -> cfblk6/1
  cfblk6/1 -> cfblk15/1
  cfblk11/1 -> cfblk17/1
  cfblk5/1 -> cfblk4/1
  cfblk13/1 -> cfblk16/1
  cfblk9/1 -> cfblk2/1
  cfblk14/1 -> cfblk3/2

== system sampleModel20/cfblk77/cfblk10/cfblk7/cfblk8 ==
  cfblk1 : Inport
  cfblk6 : Inport  Port=2
  cfblk7 : Inport  Port=3
  cfblk3 : Trigonometry
  cfblk4 : Sum  Inputs=|++
  cfblk5 : Assignment  DiagnosticForDimensions=Warning  IndexOptions=Index vector (dialog)  Indices=1  OutputSizes=1
  cfblk2 : Outport
  cfblk8 : Outport  Port=2
  wires:
  cfblk5/1 -> cfblk2/1
  cfblk7/1 -> cfblk3/1
  cfblk1/1 -> cfblk8/1
  cfblk6/1 -> cfblk4/1
  cfblk3/1 -> cfblk4/2
  cfblk4/1 -> cfblk5/1, cfblk5/2

== system sampleModel20/cfblk77/cfblk10/cfblk7/cfblk9 ==
  cfblk1 : Inport
  cfblk8 : Inport  Port=2
  cfblk9 : Inport  Port=3
  cfblk10 : Inport  Port=4
  cfblk11 : Inport  Port=5
  cfblk12 : Inport  Port=6
  cfblk3 : DotProduct  InputSameDT=on  OutDataTypeStr=Inherit: Inherit via internal rule
  cfblk4 : Math  Operator=mod  SaturateOnIntegerOverflow=on
  cfblk5 : Sum  Inputs=|++
  cfblk6 : Trigonometry
  cfblk7 : Squeeze
  cfblk2 : Outport
  cfblk13 : Outport  Port=2
  cfblk14 : Outport  Port=3
  cfblk15 : Outport  Port=4
  cfblk16 : Outport  Port=5
  wires:
  cfblk9/1 -> cfblk2/1
  cfblk6/1 -> cfblk14/1
  cfblk5/1 -> cfblk13/1
  cfblk1/1 -> cfblk5/1
  cfblk4/1 -> cfblk5/2
  cfblk10/1 -> cfblk7/1
  cfblk8/1 -> cfblk16/1, cfblk3/2
  cfblk3/1 -> cfblk6/1
  cfblk11/1 -> cfblk3/1, cfblk15/1
  cfblk12/1 -> cfblk4/1
  cfblk7/1 -> cfblk4/2

== system sampleModel20/cfblk77/cfblk4/cfblk5/cfblk3 ==
  cfblk1 : Inport
  cfblk7 : Inport  Port=2
  cfblk8 : Inport  Port=3
  cfblk9 : Inport  Port=4
  cfblk10 : Inport  Port=5
  cfblk11 : Inport  Port=6
  cfblk12 : Inport  Port=7
  cfblk3 : Polyval  Coefs=[ +2.081618890e-019, -1.441693666e-014, +4.719686976e-010, -8.536869453e-006, +1.621573104e-001, -8.087801117e+001 ]
  cfblk4 : UnaryMinus
  cfblk5 : Sum  Inputs=--
  cfblk6 : Signum
  cfblk2 : Outport
  cfblk13 : Outport  Port=2
  wires:
  cfblk1/1 -> cfblk3/1
  cfblk9/1 -> cfblk6/1
  cfblk8/1 -> cfblk2/1
  cfblk10/1 -> cfblk13/1
  cfblk12/1 -> cfblk4/1
  cfblk4/1 -> cfblk5/1
  cfblk7/1 -> cfblk5/2

== system sampleModel20/cfblk77/cfblk4/cfblk5/cfblk4 ==
  cfblk1 : Inport
  cfblk4 : Inport  Port=2
  cfblk5 : Inport  Port=3
  cfblk6 : Inport  Port=4
  cfblk7 : Inport  Port=5
  cfblk8 : Inport  Port=6
  cfblk9 : Inport  Port=7
  cfblk3 : PermuteDimensions
  cfblk2 : Outport
  cfblk10 : Outport  Port=2
  cfblk11 : Outport  Port=3
  wires:
  cfblk4/1 -> cfblk10/1
  cfblk5/1 -> cfblk3/1
  cfblk1/1 -> cfblk2/1
  cfblk6/1 -> cfblk11/1

== system sampleModel20/cfblk77/cfblk4/cfblk5/cfblk5 ==
  cfblk1 : Inport
  cfblk12 : Inport  Port=2
  cfblk13 : Inport  Port=3
  cfblk14 : Inport  Port=4
  cfblk15 : Inport  Port=5
  cfblk10 : Bias  Bias=[-348475839.320386]
  cfblk11 : Sqrt  SaturateOnIntegerOverflow=on
  cfblk16 : Delay  SampleTime=1
  cfblk17 : Delay  SampleTime=1
  cfblk3 : Trigonometry
  cfblk4 : ComplexToMagnitudeAngle
  cfblk5 : Trigonometry
  cfblk6 : Assignment  DiagnosticForDimensions=Warning  IndexOptions=Index vector (dialog)  Indices=1  OutputSizes=1
  cfblk7 : Sqrt  SaturateOnIntegerOverflow=on
  cfblk8 : simulink/Math Operations/MinMax Running Resettable  Function=min  vinit=0.0
  cfblk9 : Sum  Inputs=+
  cfblk2 : Outport
  wires:
  cfblk1/1 -> cfblk2/1
  cfblk3/1 -> cfblk7/1
  cfblk13/1 -> cfblk9/1
  cfblk10/1 -> cfblk6/1
  cfblk9/1 -> cfblk4/1
  cfblk15/1 -> cfblk8/1
  cfblk14/1 -> cfblk11/1
  cfblk5/1 -> cfblk8/2
  cfblk12/1 -> cfblk10/1
  cfblk7/1 -> cfblk6/2
  cfblk6/1 -> cfblk16/1
  cfblk16/1 -> cfblk3/1
  cfblk8/1 -> cfblk17/1
  cfblk17/1 -> cfblk5/1

== system sampleModel20/cfblk77/cfblk4/cfblk5/cfblk6 ==
  cfblk1 : Inport
  cfblk11 : Inport  Port=2
  cfblk12 : Inport  Port=3
  cfblk13 : Inport  Port=4
  cfblk10 : Reshape
  cfblk17 : Delay  SampleTime=1
  cfblk3 : simulink/Discrete/Transfer Fcn First Order  PoleZ=0.95  ICPrevOutput=0.0  DoSatur=off
  cfblk4 : Reshape
  cfblk5 : UnaryMinus
  cfblk6 : Assignment  DiagnosticForDimensions=Warning  IndexOptions=Index vector (dialog)  Indices=1  OutputSizes=1
  cfblk7 : ComplexToMagnitudeAngle
  cfblk8 : Product
  cfblk9 : Sum  Inputs=+-
  cfblk2 : Outport
  cfblk14 : Outport  Port=2
  cfblk15 : Outport  Port=3
  cfblk16 : Outport  Port=4
  wires:
  cfblk13/1 -> cfblk6/1
  cfblk11/1 -> cfblk16/1
  cfblk10/1 -> cfblk9/1
  cfblk12/1 -> cfblk7/1
  cfblk7/1 -> cfblk2/1
  cfblk5/1 -> cfblk10/1, cfblk14/1
  cfblk7/2 -> cfblk15/1
  cfblk1/1 -> cfblk8/2, cfblk6/2
  cfblk4/1 -> cfblk3/1
  cfblk6/1 -> cfblk4/1
  cfblk3/1 -> cfblk5/1
  cfblk8/1 -> cfblk9/2
  cfblk9/1 -> cfblk17/1
  cfblk17/1 -> cfblk8/1

== system sampleModel20/cfblk77/cfblk4/cfblk6/cfblk7 ==
  cfblk1 : Inport
  cfblk7 : Inport  Port=2
  cfblk3 : Reshape
  cfblk4 : PermuteDimensions
  cfblk5 : Product  Inputs=*
  cfblk6 : Product  Inputs=*
  cfblk8 : Delay  SampleTime=1
  cfblk2 : Outport
  wires:
  cfblk7/1 -> cfblk3/1
  cfblk4/1 -> cfblk6/1
  cfblk5/1 -> cfblk2/1
  cfblk3/1 -> cfblk5/1
  cfblk6/1 -> cfblk8/1
  cfblk8/1 -> cfblk4/1

== system sampleModel20/cfblk77/cfblk4/cfblk6/cfblk8 ==
  cfblk1 : Inport
  cfblk8 : Inport  Port=2
  cfblk9 : Inport  Port=3
  cfblk10 : Inport  Port=4
  cfblk11 : Inport  Port=5
  cfblk12 : Inport  Port=6
  cfblk13 : Inport  Port=7
  cfblk3 : simulink/Discrete/Transfer Fcn First Order  PoleZ=0.95  ICPrevOutput=0.0  DoSatur=off
  cfblk4 : Sqrt  Operator=rSqrt  AlgorithmType=Newton-Raphson  SaturateOnIntegerOverflow=on
  cfblk5 : Sum  Inputs=|++
  cfblk6 : ComplexToRealImag
  cfblk7 : simulink/Math Operations/MinMax Running Resettable  Function=min  vinit=0.0
  cfblk2 : Outport
  cfblk14 : Outport  Port=2
  cfblk15 : Outport  Port=3
  wires:
  cfblk3/1 -> cfblk15/1
  cfblk9/1 -> cfblk7/1
  cfblk13/1 -> cfblk6/1
  cfblk1/1 -> cfblk5/1
  cfblk8/1 -> cfblk2/1
  cfblk7/1 -> cfblk14/1
  cfblk4/1 -> cfblk7/2
  cfblk11/1 -> cfblk3/1
  cfblk10/1 -> cfblk5/2
  cfblk12/1 -> cfblk4/1

== system sampleModel20/cfblk77/cfblk4/cfblk6/cfblk9 ==
  cfblk1 : Inport
  cfblk9 : Inport  Port=2
  cfblk10 : Inport  Port=3
  cfblk11 : Inport  Port=4
  cfblk12 : Inport  Port=5
  cfblk13 : Inport  Port=6
  cfblk14 : Inport  Port=7
  cfblk15 : Inport  Port=8
  cfblk3 : Squeeze
  cfblk4 : UnaryMinus
  cfblk5 : Sqrt  Operator=rSqrt  AlgorithmType=Newton-Raphson  SaturateOnIntegerOverflow=on
  cfblk6 : Sum  Inputs=+-
  cfblk7 : Polyval  Coefs=[ +2.081618890e-019, -1.441693666e-014, +4.719686976e-010, -8.536869453e-006, +1.621573104e-001, -8.087801117e+001 ]
  cfblk8 : Gain  Gain=[296642361.786018]
  cfblk2 : Outport
  cfblk16 : Outport  Port=2
  cfblk17 : Outport  Port=3
  wires:
  cfblk9/1 -> cfblk4/1
  cfblk4/1 -> cfblk5/1
  cfblk8/1 -> cfblk7/1
  cfblk13/1 -> cfblk3/1
  cfblk3/1 -> cfblk2/1
  cfblk12/1 -> cfblk16/1
  cfblk11/1 -> cfblk17/1
  cfblk10/1 -> cfblk8/1
  cfblk5/1 -> cfblk6/1
  cfblk15/1 -> cfblk6/2

== system sampleModel20/cfblk77/cfblk5/cfblk10/cfblk10 ==
  cfblk1 : Inport
  cfblk9 : Inport  Port=2
  cfblk10 : Inport  Port=3
  cfblk11 : Inport  Port=4
  cfblk12 : Inport  Port=5
  cfblk13 : Inport  Port=6
  cfblk14 : Inport  Port=7
  cfblk15 : Inport  Port=8
  cfblk17 : Delay  SampleTime=1
  cfblk3 : Delay  ShowEnablePort=on  SampleTime=1
      settings: InputPortMap=u0,e6
  cfblk4 : Bias  Bias=[-232983956.006925]
  cfblk5 : ComplexToMagnitudeAngle
  cfblk6 : ComplexToMagnitudeAngle
  cfblk7 : Sum
  cfblk8 : ComplexToRealImag
  cfblk2 : Outport
  cfblk16 : Outport  Port=2
  wires:
  cfblk7/1 -> cfblk6/1
  cfblk9/1 -> cfblk8/1
  cfblk8/1 -> cfblk3/1
  cfblk13/1 -> cfblk7/1
  cfblk3/1 -> cfblk16/1
  cfblk10/1 -> cfblk2/1
  cfblk8/2 -> cfblk3/2
  cfblk4/1 -> cfblk5/1
  cfblk5/1 -> cfblk7/2
  cfblk6/1 -> cfblk17/1
  cfblk17/1 -> cfblk4/1

== system sampleModel20/cfblk77/cfblk5/cfblk10/cfblk11 ==
  cfblk1 : Inport
  cfblk11 : Inport  Port=2
  cfblk12 : Inport  Port=3
  cfblk10 : Reshape
  cfblk14 : Delay  SampleTime=1
  cfblk3 : DiscreteStateSpace
  cfblk4 : Assignment  DiagnosticForDimensions=Warning  IndexOptions=Index vector (dialog)  Indices=1  OutputSizes=1
  cfblk5 : Sum  Inputs=|++
  cfblk6 : Bias  Bias=[750516942.221212]
  cfblk7 : Assignment  DiagnosticForDimensions=Warning  IndexOptions=Index vector (dialog)  Indices=1  OutputSizes=1
  cfblk8 : Sum  Inputs=+-
  cfblk9 : Reshape
  cfblk2 : Outport
  cfblk13 : Outport  Port=2
  wires:
  cfblk4/1 -> cfblk6/1, cfblk14/1
  cfblk3/1 -> cfblk7/1
  cfblk6/1 -> cfblk10/1
  cfblk12/1 -> cfblk8/1
  cfblk8/1 -> cfblk3/1
  cfblk7/1 -> cfblk4/1
  cfblk11/1 -> cfblk8/2
  cfblk9/1 -> cfblk4/2, cfblk2/1
  cfblk10/1 -> cfblk13/1
  cfblk1/1 -> cfblk5/1, cfblk7/2
  cfblk5/1 -> cfblk9/1
  cfblk14/1 -> cfblk5/2

== system sampleModel20/cfblk77/cfblk5/cfblk10/cfblk12 ==
  cfblk1 : Inport
  cfblk5 : Inport  Port=2
  cfblk6 : Inport  Port=3
  cfblk3 : Sqrt  Operator=rSqrt  AlgorithmType=Newton-Raphson  SaturateOnIntegerOverflow=on
  cfblk4 : Trigonometry
  cfblk2 : Outport
  cfblk7 : Outport  Port=2
  wires:
  cfblk5/1 -> cfblk7/1
  cfblk1/1 -> cfblk3/1
  cfblk3/1 -> cfblk2/1
  cfblk6/1 -> cfblk4/1

== system sampleModel20/cfblk77/cfblk5/cfblk10/cfblk13 ==
  cfblk1 : Inport
  cfblk9 : Inport  Port=2
  cfblk3 : simulink/Discrete/Tapped Delay  vinit=0.0  samptime=-1  NumDelays=1  DelayOrder=Oldest  includeCurrent=off
  cfblk4 : simulink/Discrete/Difference  ICPrevInput=0.0  OutMin=[]  OutMax=[]  OutDataTypeStr=Inherit: Inherit via back propagation  OutDataType=fixdt(1, 16)  OutScaling=2^-10  DoSatur=off
  cfblk5 : Trigonometry
  cfblk6 : Polyval  Coefs=[ +2.081618890e-019, -1.441693666e-014, +4.719686976e-010, -8.536869453e-006, +1.621573104e-001, -8.087801117e+001 ]
  cfblk7 : Trigonometry
  cfblk8 : ComplexToRealImag
  cfblk2 : Outport
  cfblk10 : Outport  Port=2
  wires:
  cfblk1/1 -> cfblk2/1
  cfblk7/1 -> cfblk3/1
  cfblk6/1 -> cfblk10/1
  cfblk9/1 -> cfblk8/1
  cfblk4/1 -> cfblk7/1
  cfblk5/1 -> cfblk4/1
  cfblk8/1 -> cfblk6/1
  cfblk8/2 -> cfblk5/1

== system sampleModel20/cfblk77/cfblk5/cfblk10/cfblk9 ==
  cfblk1 : Inport
  cfblk9 : Inport  Port=2
  cfblk10 : Inport  Port=3
  cfblk11 : Inport  Port=4
  cfblk12 : Inport  Port=5
  cfblk13 : Inport  Port=6
  cfblk3 : Abs
  cfblk4 : MinMax  Function=max
  cfblk5 : Abs
  cfblk6 : Sqrt  SaturateOnIntegerOverflow=on
  cfblk7 : Signum
  cfblk8 : Squeeze
  cfblk2 : Outport
  cfblk14 : Outport  Port=2
  wires:
  cfblk8/1 -> cfblk2/1
  cfblk7/1 -> cfblk14/1
  cfblk1/1 -> cfblk5/1
  cfblk9/1 -> cfblk8/1
  cfblk11/1 -> cfblk4/1
  cfblk12/1 -> cfblk3/1
  cfblk10/1 -> cfblk7/1
  cfblk4/1 -> cfblk6/1

== system sampleModel20/cfblk77/cfblk5/cfblk8/cfblk10 ==
  cfblk1 : Inport
  cfblk10 : Inport  Port=2
  cfblk11 : Inport  Port=3
  cfblk12 : Inport  Port=4
  cfblk13 : Inport  Port=5
  cfblk14 : Inport  Port=6
  cfblk15 : Inport  Port=7
  cfblk18 : Delay  SampleTime=1
  cfblk3 : Squeeze
  cfblk4 : ComplexToRealImag
  cfblk5 : Trigonometry
  cfblk6 : Signum
  cfblk7 : Gain  Gain=[991233980.870795]
  cfblk8 : Gain  Gain=[-944657958.672463]
  cfblk9 : Assignment  DiagnosticForDimensions=Warning  IndexOptions=Index vector (dialog)  Indices=1  OutputSizes=1
  cfblk2 : Outport
  cfblk16 : Outport  Port=2
  cfblk17 : Outport  Port=3
  wires:
  cfblk1/1 -> cfblk5/1
  cfblk5/1 -> cfblk16/1
  cfblk4/1 -> cfblk6/1
  cfblk15/1 -> cfblk3/1
  cfblk14/1 -> cfblk8/1
  cfblk12/1 -> cfblk9/1
  cfblk7/1 -> cfblk17/1
  cfblk4/2 -> cfblk9/2
  cfblk13/1 -> cfblk7/1
  cfblk6/1 -> cfblk2/1
  cfblk9/1 -> cfblk18/1
  cfblk18/1 -> cfblk4/1

== system sampleModel20/cfblk77/cfblk5/cfblk8/cfblk11 ==
  cfblk1 : Inport
  cfblk8 : Inport  Port=2
  cfblk9 : Inport  Port=3
  cfblk10 : Inport  Port=4
  cfblk11 : Inport  Port=5
  cfblk12 : Inport  Port=6
  cfblk13 : Inport  Port=7
  cfblk3 : simulink/Discrete/Transfer Fcn First Order  PoleZ=0.95  ICPrevOutput=0.0  DoSatur=off
  cfblk4 : MinMax  Inputs=2
  cfblk5 : PermuteDimensions
  cfblk6 : ComplexToMagnitudeAngle
  cfblk7 : ComplexToMagnitudeAngle
  cfblk2 : Outport
  cfblk14 : Outport  Port=2
  cfblk15 : Outport  Port=3
  wires:
  cfblk9/1 -> cfblk3/1
  cfblk8/1 -> cfblk7/1
  cfblk10/1 -> cfblk2/1
  cfblk11/1 -> cfblk14/1
  cfblk6/1 -> cfblk5/1
  cfblk6/2 -> cfblk4/1
  cfblk4/1 -> cfblk15/1
  cfblk3/1 -> cfblk6/1
  cfblk12/1 -> cfblk4/2

== system sampleModel20/cfblk77/cfblk5/cfblk8/cfblk7 ==
  cfblk1 : Inport
  cfblk9 : Inport  Port=2
  cfblk10 : Inport  Port=3
  cfblk11 : Inport  Port=4
  cfblk12 : Inport  Port=5
  cfblk13 : Inport  Port=6
  cfblk3 : Signum
  cfblk4 : Product  Inputs=**
  cfblk5 : Abs
  cfblk6 : Polyval  Coefs=[ +2.081618890e-019, -1.441693666e-014, +4.719686976e-010, -8.536869453e-006, +1.621573104e-001, -8.087801117e+001 ]
  cfblk7 : ComplexToRealImag
  cfblk8 : Product
  cfblk2 : Outport
  cfblk14 : Outport  Port=2
  cfblk15 : Outport  Port=3
  cfblk16 : Outport  Port=4
  wires:
  cfblk1/1 -> cfblk2/1
  cfblk10/1 -> cfblk7/1
  cfblk13/1 -> cfblk3/1
  cfblk8/1 -> cfblk14/1
  cfblk4/1 -> cfblk15/1
  cfblk9/1 -> cfblk6/1
  cfblk7/1 -> cfblk5/1
  cfblk6/1 -> cfblk16/1
  cfblk12/1 -> cfblk8/1
  cfblk3/1 -> cfblk4/1
  cfblk7/2 -> cfblk8/2
  cfblk11/1 -> cfblk4/2

== system sampleModel20/cfblk77/cfblk5/cfblk8/cfblk8 ==
  cfblk1 : Inport
  cfblk7 : Inport  Port=2
  cfblk8 : Inport  Port=3
  cfblk9 : Inport  Port=4
  cfblk10 : Inport  Port=5
  cfblk11 : Inport  Port=6
  cfblk12 : Inport  Port=7
  cfblk3 : Sqrt  Operator=rSqrt  AlgorithmType=Newton-Raphson  SaturateOnIntegerOverflow=on
  cfblk4 : Reshape
  cfblk5 : Rounding
  cfblk6 : Sum  Inputs=|++
  cfblk2 : Outport
  cfblk13 : Outport  Port=2
  wires:
  cfblk8/1 -> cfblk2/1
  cfblk10/1 -> cfblk4/1
  cfblk9/1 -> cfblk5/1
  cfblk11/1 -> cfblk3/1
  cfblk3/1 -> cfblk13/1
  cfblk1/1 -> cfblk6/1
  cfblk7/1 -> cfblk6/2

== system sampleModel20/cfblk77/cfblk5/cfblk8/cfblk9 ==
  cfblk1 : Inport
  cfblk6 : Inport  Port=2
  cfblk7 : Inport  Port=3
  cfblk8 : Inport  Port=4
  cfblk9 : Inport  Port=5
  cfblk10 : Inport  Port=6
  cfblk11 : Inport  Port=7
  cfblk12 : Inport  Port=8
  cfblk3 : Assignment  DiagnosticForDimensions=Warning  IndexOptions=Index vector (dialog)  Indices=1  OutputSizes=1
  cfblk4 : UnaryMinus
  cfblk5 : Sqrt  Operator=rSqrt  AlgorithmType=Newton-Raphson  SaturateOnIntegerOverflow=on
  cfblk2 : Outport
  cfblk13 : Outport  Port=2
  cfblk14 : Outport  Port=3
  cfblk15 : Outport  Port=4
  wires:
  cfblk1/1 -> cfblk5/1
  cfblk7/1 -> cfblk3/1
  cfblk9/1 -> cfblk3/2
  cfblk11/1 -> cfblk4/1
  cfblk8/1 -> cfblk15/1
  cfblk4/1 -> cfblk14/1
  cfblk10/1 -> cfblk13/1
  cfblk5/1 -> cfblk2/1

== system sampleModel20/cfblk77/cfblk5/cfblk9/cfblk10 ==
  cfblk1 : Inport
  cfblk9 : Inport  Port=2
  cfblk10 : Inport  Port=3
  cfblk11 : Inport  Port=4
  cfblk12 : Inport  Port=5
  cfblk13 : Inport  Port=6
  cfblk14 : Inport  Port=7
  cfblk15 : Inport  Port=8
  cfblk3 : MinMax  Function=max
  cfblk4 : Sum  Inputs=+-
  cfblk5 : Math  Operator=mod  SaturateOnIntegerOverflow=on
  cfblk6 : Product
  cfblk7 : simulink/Math Operations/Slider Gain  gain=1  low=0  high=2
  cfblk8 : Sqrt  SaturateOnIntegerOverflow=on
  cfblk2 : Outport
  wires:
  cfblk7/1 -> cfblk3/1
  cfblk14/1 -> cfblk5/1
  cfblk12/1 -> cfblk7/1
  cfblk11/1 -> cfblk8/1
  cfblk13/1 -> cfblk4/1
  cfblk4/1 -> cfblk5/2
  cfblk9/1 -> cfblk2/1
  cfblk10/1 -> cfblk6/1
  cfblk8/1 -> cfblk4/2
  cfblk3/1 -> cfblk6/2

== system sampleModel20/cfblk77/cfblk5/cfblk9/cfblk11 ==
  cfblk1 : Inport
  cfblk8 : Inport  Port=2
  cfblk9 : Inport  Port=3
  cfblk10 : Inport  Port=4
  cfblk11 : Inport  Port=5
  cfblk14 : Delay  SampleTime=1
  cfblk3 : Sqrt  Operator=rSqrt  AlgorithmType=Newton-Raphson  SaturateOnIntegerOverflow=on
  cfblk4 : MinMax  Function=max  Inputs=2
  cfblk5 : Polyval  Coefs=[ +2.081618890e-019, -1.441693666e-014, +4.719686976e-010, -8.536869453e-006, +1.621573104e-001, -8.087801117e+001 ]
  cfblk6 : Gain  Gain=[251698679.866094]
  cfblk7 : Polyval  Coefs=[ +2.081618890e-019, -1.441693666e-014, +4.719686976e-010, -8.536869453e-006, +1.621573104e-001, -8.087801117e+001 ]
  cfblk2 : Outport
  cfblk12 : Outport  Port=2
  cfblk13 : Outport  Port=3
  wires:
  cfblk3/1 -> cfblk2/1
  cfblk10/1 -> cfblk3/1
  cfblk9/1 -> cfblk12/1
  cfblk11/1 -> cfblk13/1
  cfblk5/1 -> cfblk7/1
  cfblk1/1 -> cfblk4/1
  cfblk8/1 -> cfblk6/1
  cfblk6/1 -> cfblk4/2
  cfblk7/1 -> cfblk14/1
  cfblk14/1 -> cfblk5/1

== system sampleModel20/cfblk77/cfblk5/cfblk9/cfblk12 ==
  cfblk1 : Inport
  cfblk5 : Inport  Port=2
  cfblk6 : Inport  Port=3
  cfblk7 : Inport  Port=4
  cfblk3 : Signum
  cfblk4 : Sum  Inputs=|++
  cfblk2 : Outport
  wires:
  cfblk1/1 -> cfblk4/1
  cfblk3/1 -> cfblk2/1
  cfblk6/1 -> cfblk3/1
  cfblk5/1 -> cfblk4/2
